simulink model "feasibility"  (Simulink 8.1)
settings: Solver=ode45  StartTime=0.0  StopTime=10.0  RelTol=1e-3
values from neighbouring files (symbols this model uses):
  E = 1.5    [feasibility_setup.m]
  g = -100    [feasibility_setup.m]
libraries: goal x1, Numerical x1
settings Model: Creator=dejanira  LastModifiedBy=dejanira
settings DataIOCC: SignalLoggingSaveFormat=Dataset
settings OptimizationCC: ExpressionDepthLimit=128
settings DebuggingCC: FcnCallInpInsideContextMsg=EnableAllAsError
settings GRTTargetCC: CombineOutputUpdateFcns=on  GRTInterface=off

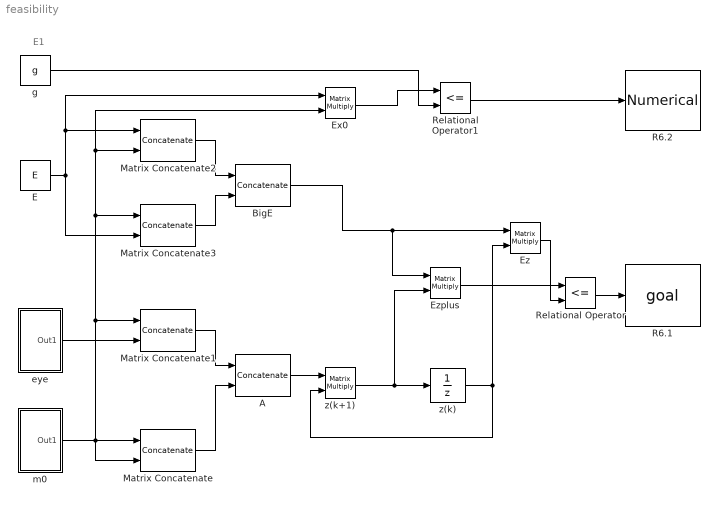
== system feasibility ==
  note: E1
  A : Concatenate  Mode=Multidimensional array
  BigE : Concatenate  Mode=Multidimensional array
  E : Constant  Value=E
  Ex0 : Product  Multiplication=Matrix(*)
  Ez : Product  Multiplication=Matrix(*)
  Ezplus : Product  Multiplication=Matrix(*)
  Matrix Concatenate{,1..3} (4 alike) : Concatenate  Mode=Multidimensional array  ConcatenateDimension=2
  R6.1 : goal/goal  SystemSampleTime=-1
  R6.2 : Numerical/Numerical  SystemSampleTime=-1
  Relational Operator : RelationalOperator  Operator=<=  OutDataTypeStr=boolean
  Relational Operator1 : RelationalOperator  Operator=<=  OutDataTypeStr=boolean
  eye : Subsystem  mask(eye){}
  g : Constant  Value=g
  m0 : Subsystem  mask(m0){}
  z(k) : UnitDelay  InitialCondition=[1;0.5]  SampleTime=-1
  z(k+1) : Product  Multiplication=Matrix(*)
  wires:
  Matrix Concatenate1/1 -> A/1
  Matrix Concatenate/1 -> A/2
  A/1 -> z(k+1)/1
  z(k)/1 -> Ez/2, z(k+1)/2
  z(k+1)/1 -> Ezplus/2, z(k)/1
  m0/1(Out1) -> Ex0/2, Matrix Concatenate2/2, Matrix Concatenate3/1, Matrix Concatenate1/1, Matrix Concatenate/2, Matrix Concatenate/1
  E/1 -> Ex0/1, Matrix Concatenate2/1, Matrix Concatenate3/2
  Matrix Concatenate2/1 -> BigE/1
  Matrix Concatenate3/1 -> BigE/2
  BigE/1 -> Ezplus/1, Ez/1
  Ez/1 -> Relational Operator/2
  Ezplus/1 -> Relational Operator/1
  Relational Operator/1 -> R6.1/1
  Relational Operator1/1 -> R6.2/1
  Ex0/1 -> Relational Operator1/1
  g/1 -> Relational Operator1/2
  eye/1(Out1) -> Matrix Concatenate1/2

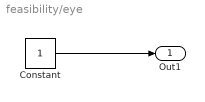
== system feasibility/eye ==
  Constant : Constant
  Out1 : Outport
  wires:
  Constant/1 -> Out1/1

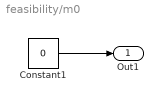
== system feasibility/m0 ==
  Constant1 : Constant  Value=0
  Out1 : Outport
  wires:
  Constant1/1 -> Out1/1
